simulink model "DhalObserverController"  (R2022a)
settings: Solver=VariableStepAuto  StartTime=0.0  StopTime=30  FixedStep=0.001  RelTol=1e-3
InitFcn:
  | params
values from neighbouring files (symbols this model uses):
  A_x = [ 0           1 ... (first row only)    [params.m]
  alpha = 1.1773*10^(6)    (= 1177300)    [params.m]
  alpha1 = 3    [params.m]
  alpha2 = 1    [params.m]
  alpha_pert = alpha - 0.35*alpha    (= 765245)    [params.m]
  B_x = [ 0 ... (first row only)    [params.m]
  beta = 5000    [params.m]
  beta_pert = beta + 0.4*beta    (= 170.78236)    [params.m]
  c = gamma/mp    (= 0.054704595186)    [params.m]
  Cinf = [1000*10^(0) 7000*10^(4)]    [params.m]
  cp_pert = cp - 0.25*cp    (= 1947.975)    [params.m]
  d = dp/mp    (= 0.25601750547)    [params.m]
  dp = 0.0468    [params.m]
  dp_pert = dp + 0.1*dp    (= 0.05148)    [params.m]
  epsilon = 0.001    [params.m]
  gamma = 0.01    [params.m]
  gamma_pert = gamma + 0.15*gamma    (= 0.0115)    [params.m]
  Kder = ( kx + kx_dot )    (= 8500)    [params.m]
  Kint = 0.01*Kprop    (= 180000.01)    [params.m]
  kp_pert = kp + 0.1*kp    (= 28671.5)    [params.m]
  kpert = 80*10^(1)    (= 800)    [params.m]
  Kprop = ( kx*kx_dot + 1 )    (= 18000001)    [params.m]
  kstate = 2*10^(1)    (= 20)    [params.m]
  kx = 450*10^(1)    (= 4500)    [params.m]
  kx_dot = 400*10^(1)    (= 4000)    [params.m]
  mp = 0.1828    [params.m]
  mp_pert = mp - 0.3*mp    (= 0.12796)    [params.m]
settings Model: Creator=Gerardo  LastModifiedBy=gerar
settings SolverCC: AlgebraicLoopSolver=TrustRegion
settings DataIOCC: LimitDataPoints=on  SaveFormat=Array  ReturnWorkspaceOutputs=off
settings OptimizationCC: BlockReduction=off  BooleanDataType=off  LifeSpan=inf
settings DebuggingCC: SaveWithParameterizedLinksMsg=none  UnderspecifiedInitializationDetection=Classic  MergeDetectMultiDrivingBlocksExec=none  SignalResolutionControl=TryResolveAllWithWarning  UnconnectedInputMsg=warning  UnconnectedOutputMsg=warning  UnconnectedLineMsg=warning  PregeneratedLibrarySubsystemCodeDiagnostic=none  SFUnexpectedBacktrackingDiag=warning  SFNoUnconditionalDefaultTransitionDiag=warning  SFExecutionAtInitializationDiag=none  SFMachineParentedDataDiag=warning  ArithmeticOperatorsInVariantConditions=warning
settings HardwareCC: ProdBitPerPointer=32  ProdBitPerSizeT=32  ProdBitPerPtrDiffT=32  ProdLargestAtomicFloat=None  ProdIntDivRoundTo=Undefined  ProdEndianess=Unspecified  ProdWordSize=32  ProdHWDeviceType=32-bit Generic  TargetUnknown=on
settings ModelReferenceCC: PropagateSignalLabelsOutOfModel=off
settings SFSimCC: SimUseLocalCustomCode=off  CustomCodeUndefinedFunction=UseInterfaceOnly
settings RTWCC: RTWUseLocalCustomCode=off
settings CodeAppCC: StateflowObjectComments=on
settings GRTTargetCC: TargetLangStandard=C89/C90 (ANSI)
settings ConfigComp: CovMetricSettings=dw  CovSaveCumulativeToWorkspaceVar=on  CovSaveSingleToWorkspaceVar=on  CovExternalEMLEnable=off  CovSFcnEnable=off

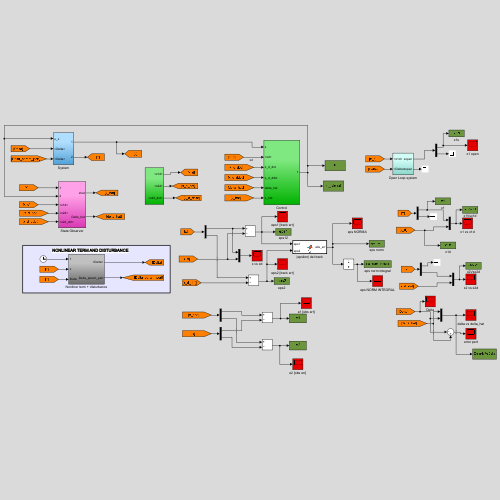
[thumbnail: Simulink's stored preview of the top-level diagram]
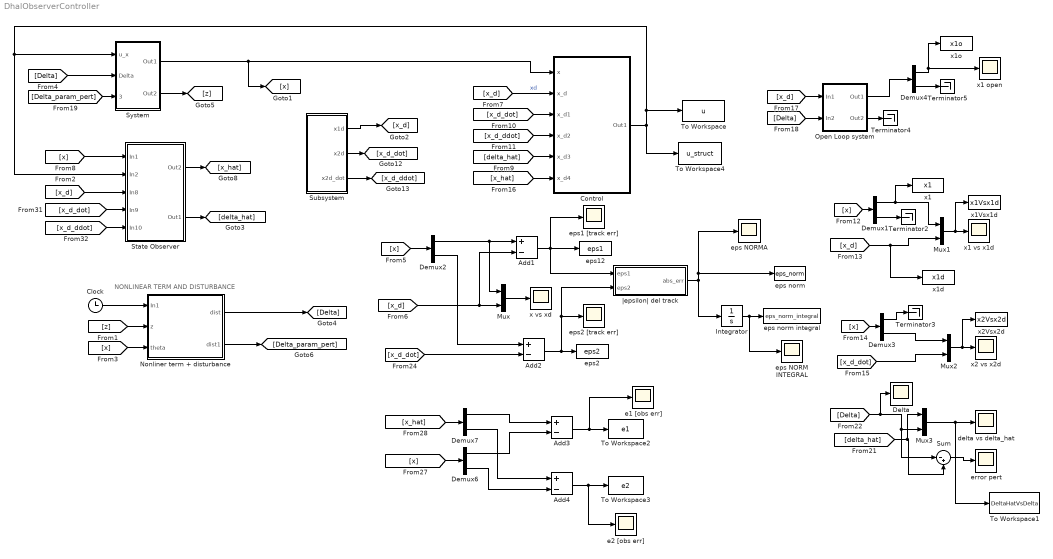
== system DhalObserverController ==
  note: NONLINEAR TERM AND DISTURBANCE
  Add{1..4} (4 alike) : Sum  Inputs=+-
  Clock : Clock
  Control : Subsystem
  Delta : Scope
  Demux{1..4,6..7} (6 alike) : Demux  Outputs=2
  Integrator : Integrator
  Mux{,1..3} (4 alike) : Mux  Inputs=2
  Nonliner term + disturbance : Subsystem
  Open Loop system : Subsystem
  State Observer : Subsystem
  Subsystem : Subsystem
  Sum : Sum  Inputs=|-+
  System : Subsystem
  Terminator{2..5} (4 alike) : Terminator
  To Workspace : ToWorkspace  VariableName=u  SaveFormat=Timeseries  SampleTime=-1
  To Workspace1 : ToWorkspace  VariableName=DeltaHatVsDelta  SaveFormat=Timeseries  SampleTime=-1
  To Workspace2 : ToWorkspace  VariableName=e1  SaveFormat=Timeseries  SampleTime=-1
  To Workspace3 : ToWorkspace  VariableName=e2  SaveFormat=Timeseries  SampleTime=-1
  To Workspace4 : ToWorkspace  VariableName=u_struct  SaveFormat=Structure With Time  SampleTime=-1
  delta vs delta_hat : Scope
  e1 [obs err] : Scope
  e2 [obs err] : Scope
  eps NORM INTEGRAL : Scope
  eps NORMA : Scope
  eps norm : ToWorkspace  VariableName=eps_norm  SaveFormat=Timeseries  SampleTime=-1
  eps norm integral : ToWorkspace  VariableName=eps_norm_integral  SaveFormat=Timeseries  SampleTime=-1
  eps1 [track err] : Scope
  eps12 : ToWorkspace  VariableName=eps1  SaveFormat=Timeseries  SampleTime=-1
  eps2 : ToWorkspace  VariableName=eps2  SaveFormat=Timeseries  SampleTime=-1
  eps2 [track err] : Scope
  error pert : Scope
  x vs xd : Scope
  x1 : ToWorkspace  VariableName=x1  SaveFormat=Structure With Time  SampleTime=-1
  x1 open : Scope
  x1 vs x1d : Scope
  x1Vsx1d : ToWorkspace  VariableName=x1Vsx1d  SaveFormat=Timeseries  SampleTime=-1
  x1d : ToWorkspace  VariableName=x1d  SaveFormat=Structure With Time  SampleTime=-1
  x1o : ToWorkspace  VariableName=x1o  SaveFormat=Structure With Time  SampleTime=-1
  x2 vs x2d : Scope
  x2Vsx2d : ToWorkspace  VariableName=x2Vsx2d  SaveFormat=Timeseries  SampleTime=-1
  |epsilon| del track : MATLAB Function  TreatAsAtomicUnit=on
  wires:
  State Observer/1(Out2) -> [x_hat]
  [Delta] -> System/2(Delta)
  Control/1(Out1) -> To Workspace/1, System/1(u_x), State Observer/2(In2), To Workspace4/1
  [x] -> State Observer/1(In1)
  [x] -> Demux2/1
  Mux/1 -> x vs xd/1
  System/1(Out1) -> [x], Control/1(x)
  Subsystem/1(x1d) -> [x_d]
  State Observer/2(Out1) -> [delta_hat]
  [Delta] -> Delta/1, Mux3/2, Sum/1
  [delta_hat] -> Mux3/1, Sum/2
  Mux3/1 -> To Workspace1/1, delta vs delta_hat/1
  Clock/1 -> Nonliner term + disturbance/1(In1)
  [x_d_dot] -> State Observer/4(In9)
  [x_d_ddot] -> State Observer/5(In10)
  [x_d] -> State Observer/3(In8)
  Nonliner term + disturbance/1(dist) -> [Delta]
  [z] -> Nonliner term + disturbance/2(z)
  System/2(Out2) -> [z]
  [x] -> Nonliner term + disturbance/3(theta)
  Demux2/1 -> Add1/1, Mux/1
  [x_d] -> Add1/2, Mux/2
  Subsystem/2(x2d) -> [x_d_dot]
  Subsystem/3(x2d_dot) -> [x_d_ddot]
  [x_d] -> Control/2(x_d)  "xd"
  [x_d_dot] -> Control/3(x_d1)
  [x_d_ddot] -> Control/4(x_d2)
  [delta_hat] -> Control/5(x_d3)
  [x_hat] -> Control/6(x_d4)
  Sum/1 -> error pert/1
  [x_d] -> x1d/1, Mux1/2
  Demux1/1 -> x1/1, Mux1/1
  Demux1/2 -> Terminator2/1
  Mux1/1 -> x1Vsx1d/1, x1 vs x1d/1
  [x] -> Demux1/1
  [x] -> Demux3/1
  Mux2/1 -> x2Vsx2d/1, x2 vs x2d/1
  [x_d_dot] -> Mux2/2
  Demux3/1 -> Terminator3/1
  Demux3/2 -> Mux2/1
  [x_d] -> Open Loop system/1(In1)
  [Delta] -> Open Loop system/2(In2)
  Open Loop system/2(Out2) -> Terminator4/1
  Open Loop system/1(Out1) -> Demux4/1
  Demux4/2 -> Terminator5/1
  Demux4/1 -> x1 open/1, x1o/1
  Add1/1 -> |epsilon| del track/1(eps1), eps1 [track err]/1, eps12/1
  Demux2/2 -> Add2/1
  [x_d_dot] -> Add2/2
  Add2/1 -> eps2 [track err]/1, |epsilon| del track/2(eps2), eps2/1
  [x] -> Demux6/1
  [x_hat] -> Demux7/1
  Demux7/1 -> Add3/1
  Demux6/1 -> Add3/2
  Add3/1 -> e1 [obs err]/1, To Workspace2/1
  Demux7/2 -> Add4/1
  Demux6/2 -> Add4/2
  Add4/1 -> e2 [obs err]/1, To Workspace3/1
  |epsilon| del track/1(abs_err) -> Integrator/1, eps NORMA/1, eps norm/1
  Integrator/1 -> eps NORM INTEGRAL/1, eps norm integral/1
  Nonliner term + disturbance/2(dist1) -> [Delta_param_pert]
  [Delta_param_pert] -> System/3(Delta1)

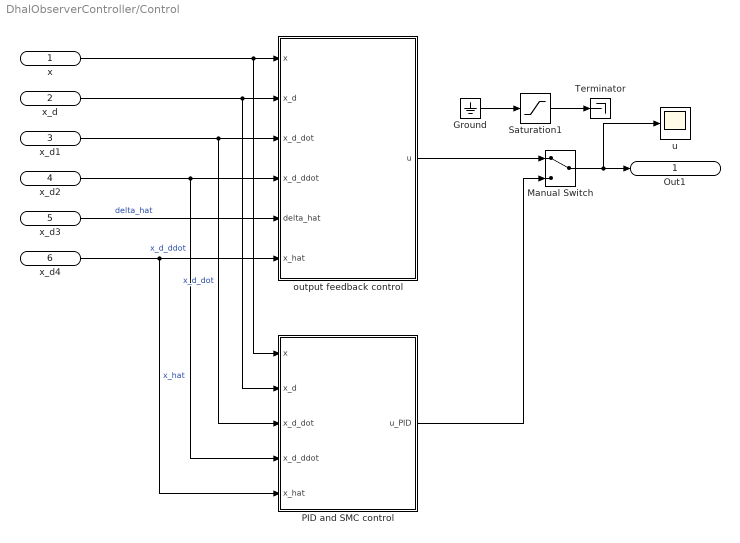
== system DhalObserverController/Control ==
  x : Inport
  x_d : Inport  Port=2
  x_d1 : Inport  Port=3
  x_d2 : Inport  Port=4
  x_d3 : Inport  Port=5
  x_d4 : Inport  Port=6
  Ground : Ground
  Manual Switch : ManualSwitch
  PID and SMC control : Subsystem
  Saturation1 : Saturate  UpperLimit=25  LowerLimit=-25
  Terminator : Terminator
  output feedback control : MATLAB Function  TreatAsAtomicUnit=on
  "u " : Scope
  Out1 : Outport  VectorParamsAs1DForOutWhenUnconnected=off
  wires:
  x/1 -> PID and SMC control/1(x), output feedback control/1(x)
  Ground/1 -> Saturation1/1
  Saturation1/1 -> Terminator/1
  x_d/1 -> PID and SMC control/2(x_d), output feedback control/2(x_d)
  x_d1/1 -> PID and SMC control/3(x_d_dot), output feedback control/3(x_d_dot)  "x_d_dot"
  x_d2/1 -> PID and SMC control/4(x_d_ddot), output feedback control/4(x_d_ddot)  "x_d_ddot"
  x_d3/1 -> output feedback control/5(delta_hat)  "delta_hat"
  x_d4/1 -> PID and SMC control/5(x_hat), output feedback control/6(x_hat)  "x_hat"
  Manual Switch/1 -> "u "/1, Out1/1
  output feedback control/1(u) -> Manual Switch/1
  PID and SMC control/1(u_PID) -> Manual Switch/2

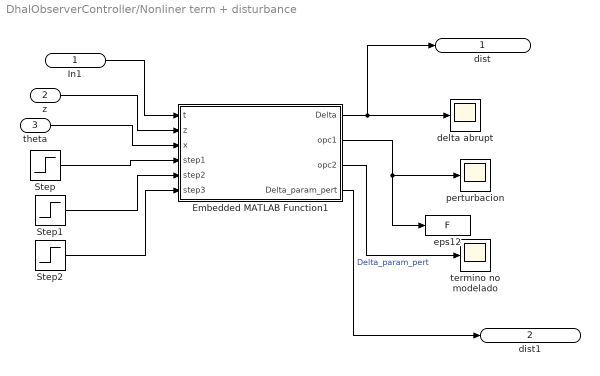
== system DhalObserverController/Nonliner term + disturbance ==
  In1 : Inport
  z : Inport  Port=2
  theta : Inport  Port=3
  Embedded MATLAB Function1 : MATLAB Function  TreatAsAtomicUnit=on
  Step : Step  Time=6  SampleTime=0
  Step1 : Step  Time=12  SampleTime=0
  Step2 : Step  Time=22  SampleTime=0
  delta abrupt : Scope
  eps12 : ToWorkspace  VariableName=F  SaveFormat=Timeseries  SampleTime=-1
  perturbacion : Scope
  termino no modelado : Scope
  dist : Outport  VectorParamsAs1DForOutWhenUnconnected=off
  dist1 : Outport  Port=2  VectorParamsAs1DForOutWhenUnconnected=off
  wires:
  Step/1 -> Embedded MATLAB Function1/4(step1)
  In1/1 -> Embedded MATLAB Function1/1(t)
  Step2/1 -> Embedded MATLAB Function1/6(step3)
  Embedded MATLAB Function1/1(Delta) -> delta abrupt/1, dist/1
  Step1/1 -> Embedded MATLAB Function1/5(step2)
  z/1 -> Embedded MATLAB Function1/2(z)
  theta/1 -> Embedded MATLAB Function1/3(x)
  Embedded MATLAB Function1/2(opc1) -> eps12/1, perturbacion/1
  Embedded MATLAB Function1/3(opc2) -> termino no modelado/1
  Embedded MATLAB Function1/4(Delta_param_pert) -> dist1/1  "Delta_param_pert"

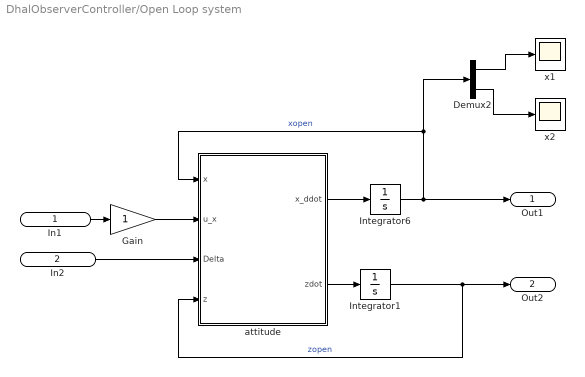
== system DhalObserverController/Open Loop system ==
  In1 : Inport
  In2 : Inport  Port=2
  Demux2 : Demux  Outputs=2
  Gain : Gain
  Integrator1 : Integrator  InitialCondition=2
  Integrator6 : Integrator  InitialCondition=[0.25; 1]
  attitude : MATLAB Function  TreatAsAtomicUnit=on
  x1 : Scope
  x2 : Scope
  Out1 : Outport  VectorParamsAs1DForOutWhenUnconnected=off
  Out2 : Outport  Port=2  VectorParamsAs1DForOutWhenUnconnected=off
  wires:
  attitude/1(x_ddot) -> Integrator6/1
  Integrator6/1 -> Demux2/1, attitude/1(x), Out1/1  "xopen"
  In1/1 -> Gain/1
  In2/1 -> attitude/3(Delta)
  Demux2/1 -> x1/1
  Demux2/2 -> x2/1
  attitude/2(zdot) -> Integrator1/1
  Integrator1/1 -> Out2/1, attitude/4(z)  "zopen"
  Gain/1 -> attitude/2(u_x)

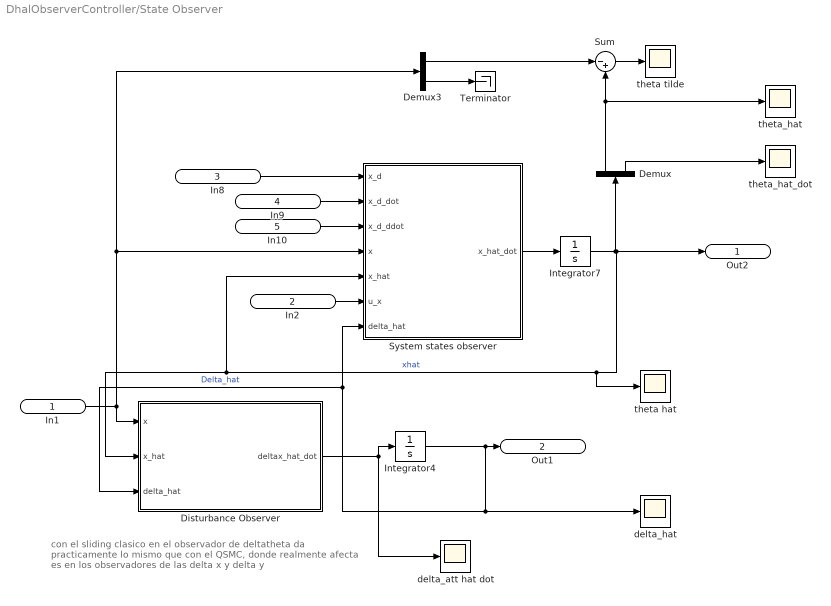
== system DhalObserverController/State Observer ==
  note: con el sliding clasico en el observador de deltatheta da
      | practicamente lo mismo que con el QSMC, donde
      | realmente afecta es en los observadores de las delta x y delta y
  In1 : Inport
  In2 : Inport  Port=2
  In8 : Inport  Port=3
  In9 : Inport  Port=4
  In10 : Inport  Port=5
  Demux : Demux  Outputs=2
  Demux3 : Demux  Outputs=2
  Disturbance Observer : MATLAB Function  TreatAsAtomicUnit=on
  Integrator4 : Integrator
  Integrator7 : Integrator  InitialCondition=[0; 0]  UpperSaturationLimit=10  LowerSaturationLimit=-10
  Sum : Sum  Inputs=|-+
  System states observer : MATLAB Function  TreatAsAtomicUnit=on
  Terminator : Terminator
  delta_att hat dot : Scope
  delta_hat : Scope
  theta hat : Scope
  theta tilde : Scope
  theta_hat : Scope
  theta_hat_dot : Scope
  Out2 : Outport  VectorParamsAs1DForOutWhenUnconnected=off
  Out1 : Outport  Port=2  VectorParamsAs1DForOutWhenUnconnected=off
  wires:
  Disturbance Observer/1(deltax_hat_dot) -> Integrator4/1, delta_att hat dot/1
  Integrator4/1 -> System states observer/7(delta_hat), Disturbance Observer/3(delta_hat), delta_hat/1, Out1/1  "Delta_hat"
  Integrator7/1 -> Out2/1, System states observer/5(x_hat), Disturbance Observer/2(x_hat), theta hat/1, Demux/1  "xhat"
  Demux/1 -> theta_hat/1, Sum/2
  Demux3/1 -> Sum/1
  Sum/1 -> theta tilde/1
  In2/1 -> System states observer/6(u_x)
  In1/1 -> Demux3/1, System states observer/4(x), Disturbance Observer/1(x)
  Demux/2 -> theta_hat_dot/1
  In9/1 -> System states observer/2(x_d_dot)
  In8/1 -> System states observer/1(x_d)
  System states observer/1(x_hat_dot) -> Integrator7/1
  In10/1 -> System states observer/3(x_d_ddot)
  Demux3/2 -> Terminator/1

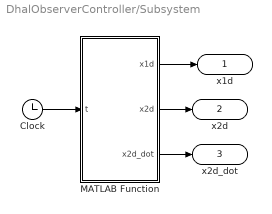
== system DhalObserverController/Subsystem ==
  Clock : Clock
  MATLAB Function : MATLAB Function  TreatAsAtomicUnit=on
  x1d : Outport  VectorParamsAs1DForOutWhenUnconnected=off
  x2d : Outport  Port=2  VectorParamsAs1DForOutWhenUnconnected=off
  x2d_dot : Outport  Port=3  VectorParamsAs1DForOutWhenUnconnected=off
  wires:
  Clock/1 -> MATLAB Function/1(t)
  MATLAB Function/1(x1d) -> x1d/1
  MATLAB Function/2(x2d) -> x2d/1
  MATLAB Function/3(x2d_dot) -> x2d_dot/1

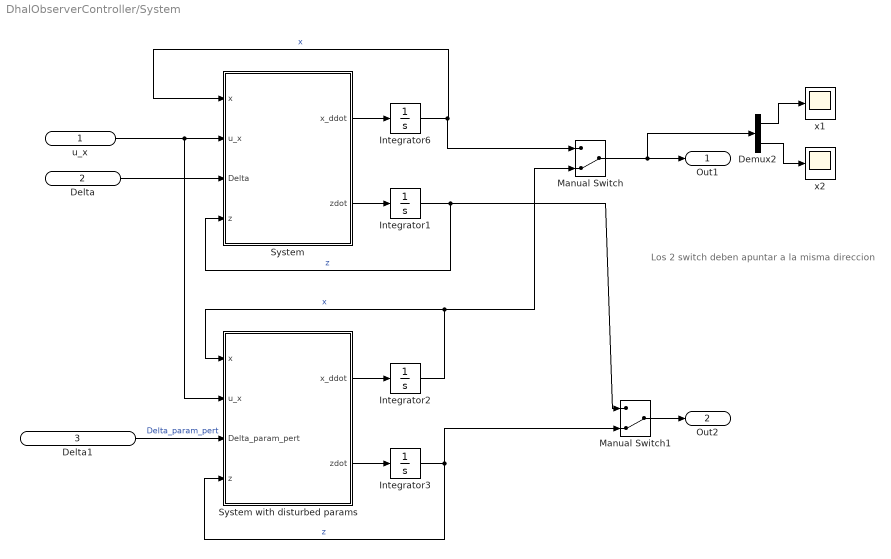
== system DhalObserverController/System ==
  note: Los 2 switch deben apuntar a la misma direccion
  u_x : Inport
  Delta : Inport  Port=2
  Delta1 : Inport  Port=3
  Demux2 : Demux  Outputs=2
  Integrator1 : Integrator  InitialCondition=2
  Integrator2 : Integrator  InitialCondition=[0.25; 1]
  Integrator3 : Integrator  InitialCondition=2
  Integrator6 : Integrator  InitialCondition=[0.25; 1]
  Manual Switch : ManualSwitch  CurrentSetting=0
  Manual Switch1 : ManualSwitch  CurrentSetting=0
  System : MATLAB Function  TreatAsAtomicUnit=on
  System with disturbed params : MATLAB Function  TreatAsAtomicUnit=on
  x1 : Scope
  x2 : Scope
  Out1 : Outport  VectorParamsAs1DForOutWhenUnconnected=off
  Out2 : Outport  Port=2  VectorParamsAs1DForOutWhenUnconnected=off
  wires:
  System/1(x_ddot) -> Integrator6/1
  Integrator6/1 -> Manual Switch/1, System/1(x)  "x"
  u_x/1 -> System with disturbed params/2(u_x), System/2(u_x)
  Delta/1 -> System/3(Delta)
  Demux2/1 -> x1/1
  Demux2/2 -> x2/1
  System/2(zdot) -> Integrator1/1
  Integrator1/1 -> System/4(z), Manual Switch1/1  "z"
  System with disturbed params/1(x_ddot) -> Integrator2/1
  System with disturbed params/2(zdot) -> Integrator3/1
  Integrator2/1 -> Manual Switch/2, System with disturbed params/1(x)  "x"
  Integrator3/1 -> Manual Switch1/2, System with disturbed params/4(z)  "z"
  Manual Switch/1 -> Demux2/1, Out1/1
  Manual Switch1/1 -> Out2/1
  Delta1/1 -> System with disturbed params/3(Delta_param_pert)  "Delta_param_pert"

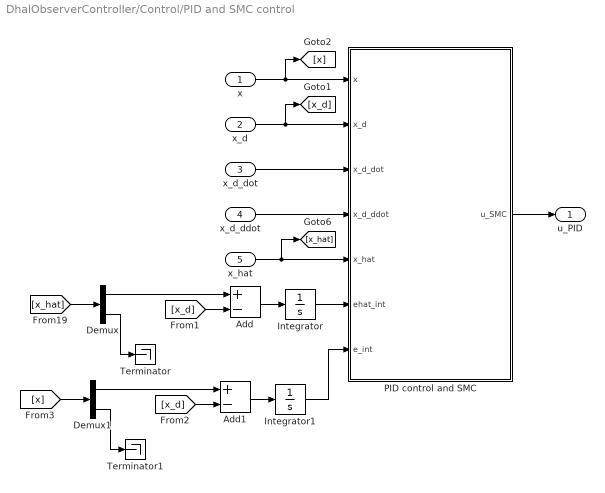
== system DhalObserverController/Control/PID and SMC control ==
  x : Inport
  x_d : Inport  Port=2
  x_d_dot : Inport  Port=3
  x_d_ddot : Inport  Port=4
  x_hat : Inport  Port=5
  Add : Sum  Inputs=+-
  Add1 : Sum  Inputs=+-
  Demux : Demux  Outputs=2
  Demux1 : Demux  Outputs=2
  Integrator : Integrator
  Integrator1 : Integrator
  PID control and SMC : MATLAB Function  TreatAsAtomicUnit=on
  Terminator : Terminator
  Terminator1 : Terminator
  u_PID : Outport
  wires:
  x/1 -> [x], PID control and SMC/1(x)
  x_d/1 -> [x_d], PID control and SMC/2(x_d)
  x_d_dot/1 -> PID control and SMC/3(x_d_dot)
  x_d_ddot/1 -> PID control and SMC/4(x_d_ddot)
  x_hat/1 -> [x_hat], PID control and SMC/5(x_hat)
  PID control and SMC/1(u_SMC) -> u_PID/1
  Add/1 -> Integrator/1
  Demux/2 -> Terminator/1
  [x_hat] -> Demux/1
  Demux/1 -> Add/1
  [x_d] -> Add/2
  Add1/1 -> Integrator1/1
  Demux1/1 -> Add1/1
  [x_d] -> Add1/2
  Demux1/2 -> Terminator1/1
  [x] -> Demux1/1
  Integrator/1 -> PID control and SMC/6(ehat_int)
  Integrator1/1 -> PID control and SMC/7(e_int)

== matlab function DhalObserverController/System/System with disturbed params ==
  data: x input; u_x input; Delta_param_pert input; z input; x_ddot output; B_x parameter; zdot output; kp_pert parameter; mp_pert parameter; cp_pert parameter; dp_pert parameter; alpha_pert parameter; beta_pert parameter
function [x_ddot, zdot] = fcn(x, u_x, Delta_param_pert, z, B_x, kp_pert, mp_pert, cp_pert, dp_pert, alpha_pert, beta_pert)

x2 = x(2,1);

%perturbed parameters:
%A_x_pert = [   0                1          ;
%            -(kp/mp + 0.2*kp/mp)  -(14208)-0.25*(14208)];

A_x_pert = [          0        ,          1          ;
             -kp_pert/mp_pert  ,  -cp_pert/mp_pert  ];

%Perturbed system
x_ddot = A_x_pert * x + B_x*( (dp_pert/mp_pert)*u_x + Delta_param_pert );
zdot = - alpha_pert * x2 - beta_pert * abs(x2)*z;
%zdot = - (alpha - 0.4*alpha) * x2 - (beta + 0.6*beta) * abs(x2)*z;

== matlab function DhalObserverController/Control/output feedback control ==
  data: x input; x_d input; x_d_dot input; x_d_ddot input; delta_hat input; x_hat input; u output; kx parameter; kx_dot parameter; A_x parameter; d parameter
function u = fcn(x, x_d, x_d_dot, x_d_ddot, delta_hat, x_hat, kx, kx_dot, A_x, d)

%compensacion de los terminos del sistema Dahl:
comp = A_x * x_hat;
           
%Con la theta estimada delta_att_hat:
%u_x = (1/d)*(- kx*( x_hat(1,1) - x_d ) - kx_dot*( x_hat(2,1) - x_d_dot) + x_d_ddot - 1*delta_hat - comp(2,1)) ;
%backstepping [final]:
u = (1/d)*(  - comp(2,1) - delta_hat + x_d_ddot - ( kx*kx_dot + 1 )*( x_hat(1,1) - x_d ) - ( kx + kx_dot )*( x_hat(2,1) - x_d_dot)   ) ;

== matlab function DhalObserverController/State Observer/Disturbance Observer ==
  data: x input; x_hat input; deltax_hat_dot output; delta_hat input; kstate parameter; kpert parameter; epsilon parameter
function deltax_hat_dot  = fcn(x, x_hat, delta_hat, kstate, kpert, epsilon)

%%%%%%%%%%%%%%%%%%%%%%%%% ORIGINAL 
%deltaAtt_hat_dot =  - 0.84*sign(theta_hat(1,1) - theta(1,1)) - 1.45*deltaAtt_hat;
%%%%%%%%%%%%%%%%%%%%%%%%% ORIGINAL 

%%%%%%%%%%%%%%%%%%%%%%%%% QSMC
ex = x_hat(1,1) - x(1,1);
%sigmax = pend*ex ;
deltax_hat_dot = - kpert*( ex/( abs(ex) + epsilon ) ) - kstate*delta_hat ;
%deltax_hat_dot = - kpert*sign(ex) - kstate*delta_hat - 0*kstate*( x(1,1) - x_d(1,1) );
%el valor de 100 entre mas grande sea mejor sigue la perturbacion
%%%%%%%%%%%%%%%%%%%%%%%%% QSMC  kstate

== matlab function DhalObserverController/State Observer/System states observer ==
  data: x_d input; x_d_dot input; x_d_ddot input; x input; x_hat input; u_x input; delta_hat input; A_x parameter; B_x parameter; Cinf parameter; kx parameter; kx_dot parameter; x_hat_dot output; d parameter
function x_hat_dot = fcn(x_d, x_d_dot, x_d_ddot, x, x_hat, u_x, delta_hat, A_x, B_x, Cinf, kx, kx_dot, d)

%compensacion:
%comp = theta_hat(1,1) + theta_hat(2,1);
%u_theta_new = - ktheta*( theta_hat(1,1) - theta_d ) - ktheta_dot*( theta_hat(2,1) - theta_d_dot ) + theta_d_ddot ;

x_hat_dot = A_x*x_hat + B_x*( d*u_x + delta_hat) - Cinf'*(x_hat(1,1) - x(1,1));



%%%%%% viejos
%theta = 1
%C2 = [200 10000]; %C2 = [2 1]; %C2 = [20 100] --- si funciona el observador del estado, no el de la pert;

%ESTE ES EL QUE ESTA PROGRAMADO
%u_theta_new = - ktheta*theta_hat(1,1) - ktheta_dot*theta_hat(2,1);
%u_theta_new = - ktheta*( theta_hat(1,1) - theta_d ) - ktheta_dot*( theta_hat(2,1) - theta_d_dot); %este es con deseado, como esta demostrado
%theta_hat_dot = A_theta*theta_hat + B_theta*( u_theta_new ) - Cinf'*(theta_hat(1,1) - theta(1,1));

%u_theta_new = - ktheta*theta_tilde_hat(1,1) - ktheta_dot*theta_tilde_hat(2,1);
%theta_tilde_hat_dot = A_theta*theta_tilde_hat + B_theta*( u_theta_new ) - Cinf'*(theta_tilde_hat(1,1) - theta_tilde_1(1,1));

%out ESTE SI FUNCIONA
%theta_hat_dot = A_theta*theta_hat + B_theta*(u_theta + deltaAtt_hat) - Cinf'*(theta_hat(1,1) - theta(1,1));

== matlab function DhalObserverController/|epsilon| del track ==
  data: eps1 input; abs_err output; eps2 input
function abs_err = fcn(eps1, eps2)

abs_err = sqrt(eps1^2 + eps2^2);

== matlab function DhalObserverController/Nonliner term + disturbance/Embedded MATLAB Function1 ==
  data: Delta output; t input; z input; x input; step1 input; step2 input; step3 input; c parameter; mp parameter; opc1 output; opc2 output; gamma parameter; Delta_param_pert output; mp_pert parameter; gamma_pert parameter
function [Delta, opc1, opc2, Delta_param_pert] = pert(t, z, x, step1, step2, step3, c, mp, gamma, mp_pert, gamma_pert)

%Original
%dist = 5*exp(-0.08*(t-0.03))*step1 + 8*exp(-0.05*(t-1))*step2 + 5.6*exp(-0.03*(t-1.3))*step3    ;

x2 = x(2,1);
dist =  0.5*exp(-0.08*(t-0.03))*step1 + 0.8*exp(-0.05*(t-1))*step2 + 0.56*exp(-0.03*(t-1.3))*step3    ;
Delta = - (gamma/mp)*sign(x2)*z - 100*(dist + 1)/(mp);

%Only for the case of variations in the parameters
Delta_param_pert = - (gamma_pert/mp_pert)*sign(x2)*z - 100*(dist + 1)/(mp_pert);

opc1 = - 100*(dist + 1)/(mp);
opc2 = - (gamma/mp)*sign(x2)*z;

== matlab function DhalObserverController/System/System ==
  data: x input; u_x input; Delta input; z input; x_ddot output; A_x parameter; B_x parameter; zdot output; alpha parameter; beta parameter; mp parameter; dp parameter
function [x_ddot, zdot] = fcn(x, u_x, Delta, z, A_x, B_x, alpha, beta, mp, dp)

x2 = x(2,1);

x_ddot = A_x * x + B_x*( (dp/mp)*u_x + Delta );
zdot = - alpha * x2 - beta * abs(x2)*z;

== matlab function DhalObserverController/Subsystem/MATLAB Function ==
  data: t input; x1d output; freq parameter; x2d output; x2d_dot output
function [x1d, x2d, x2d_dot] = fcn(t, freq)


x1d = 80*sin(freq*t);
x2d = 80*freq*cos(freq*t);
x2d_dot = - 80*freq^2*sin(freq*t);

== matlab function DhalObserverController/Open Loop system/attitude ==
  data: x input; u_x input; Delta input; z input; x_ddot output; A_x parameter; B_x parameter; zdot output; alpha parameter; beta parameter; mp parameter; dp parameter
function [x_ddot, zdot] = fcn(x, u_x, Delta, z, A_x, B_x, alpha, beta, mp, dp)

x2 = x(2,1);
%out
x_ddot = A_x * x + B_x*( (dp/mp)*u_x + Delta );
zdot = - alpha * x2 - beta * abs(x2)*z;

== matlab function DhalObserverController/Control/PID and SMC control/PID control and SMC ==
  data: x input; x_d input; x_d_dot input; x_d_ddot input; x_hat input; ehat_int input; e_int input; u_SMC output; A_x parameter; d parameter; Kprop parameter; Kder parameter; Kint parameter; alpha1 parameter; alpha2 parameter; beta parameter
function u_SMC = fcn(x, x_d, x_d_dot, x_d_ddot, x_hat, ehat_int, e_int, A_x, d, Kprop, Kder, Kint, alpha1, alpha2, beta)

% Término de compensación
comp = A_x * x_hat;

%PID control
%u_PID = (1/d)*( - Kprop * ( x_hat(1,1) - x_d ) - Kder * ( x_hat(2,1) - x_d_dot) - Kint * ehat_int - 0*comp(2,1) + 0*x_d_ddot ) ; 


%SMC de INDICON [modificado]
e1 =  x_hat(1,1) - x_d ; 
e2 =  x_hat(2,1) - x_d_dot ; 
z = ehat_int;
sigma = e1 + alpha1 * e2 + alpha2 * z ;

u_SMC = (1/d)*( - beta*sign( sigma ) - comp(2,1) + x_d_ddot ) ; 


%************************************************************************

%%%%% VIEJO:
%PD
%u_p = (1/d)*(- 35000 *( x(1,1) - x_d ) );
% u_pd = (1/d)*(- 3510000 *( x(1,1) - x_d ) - 390000*( x(2,1) - x_d_dot) )
% ; con esta funciono mas o menos
